simulink model "SFC_FF_con_osservatore"  (R2023a)
settings: Solver=VariableStepAuto  StartTime=0.0  StopTime=10.0  RelTol=1e-3
undefined symbols (not defined in the file or in its folder): A, B, C, Cu, K, Kr, L
settings Model: Creator=vince  LastModifiedBy=vince

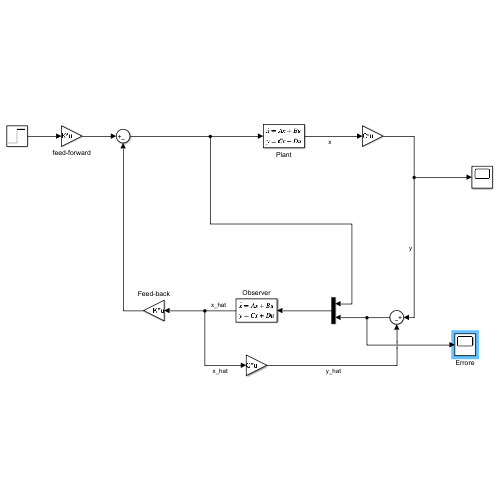
[thumbnail: Simulink's stored preview of the top-level diagram]
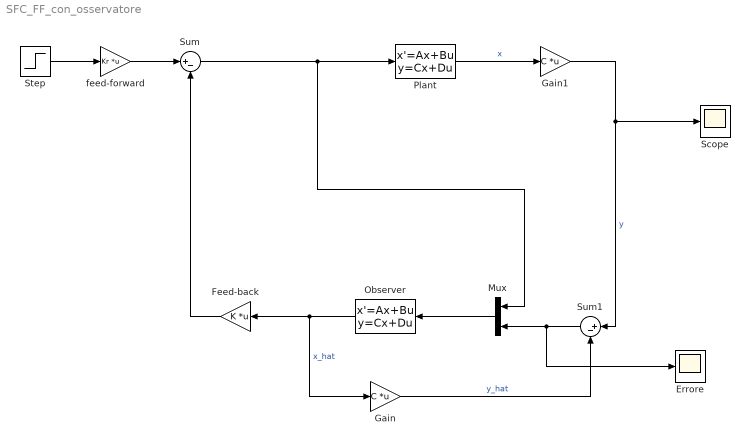
== system SFC_FF_con_osservatore ==
  Errore : Scope
  Feed-back : Gain  Gain=K  Multiplication=Matrix(K*u)
  Gain : Gain  Gain=C  Multiplication=Matrix(K*u)
  Gain1 : Gain  Gain=C  Multiplication=Matrix(K*u)
  Mux : Mux  Inputs=2
  Observer : StateSpace  A=A  B=[B L]  C=Cu  D=[0 0; 0 0]  InitialCondition=0
  Plant : StateSpace  A=A  B=B  C=Cu  D=[0 ; 0]  InitialCondition=[1 0.5]  ParameterTunability=Unconstrained
  Scope : Scope
  Step : Step  Time=0  SampleTime=0
  Sum : Sum  Inputs=|+-
  Sum1 : Sum  Inputs=|+-
  feed-forward : Gain  Gain=Kr  Multiplication=Matrix(K*u)
  wires:
  Mux/1 -> Observer/1
  Step/1 -> feed-forward/1
  feed-forward/1 -> Sum/1
  Feed-back/1 -> Sum/2
  Sum/1 -> Mux/1, Plant/1
  Plant/1 -> Gain1/1  "x"
  Gain1/1 -> Scope/1, Sum1/1  "y"
  Sum1/1 -> Errore/1, Mux/2
  Gain/1 -> Sum1/2  "y_hat"
  Observer/1 -> Gain/1, Feed-back/1  "x_hat"
